simulink model "untitled1"  (R2024b)
settings: Solver=VariableStepAuto  StartTime=0.0  StopTime=0.005  RelTol=1e-3
libraries: simulink x1
settings Model: Creator=valun  LastModifiedBy=valun

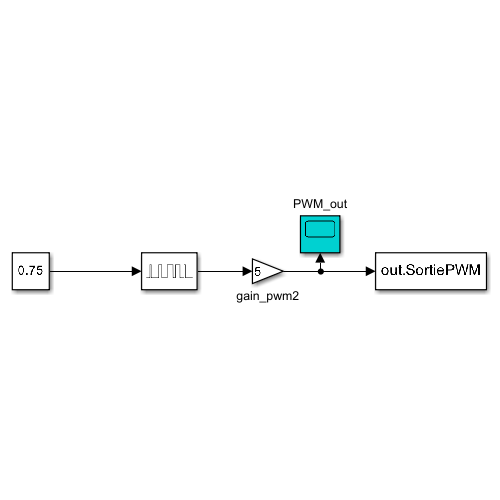
[thumbnail: Simulink's stored preview of the top-level diagram]
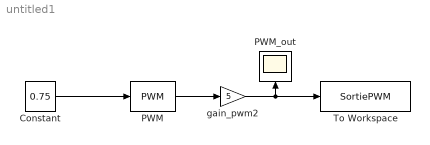
== system untitled1 ==
  Constant : Constant  Value=0.75
  PWM : simulink/Discontinuities/PWM  DisableCoverage=on  Period=0.001  InitialDelay=0  DisallowZeroDutyCycle=off  RunAtFixedTimeIntervals=off  SampleTime=0.1
  PWM_out : Scope
  To Workspace : ToWorkspace  VariableName=SortiePWM  SampleTime=-1
  gain_pwm2 : Gain  Gain=5
  wires:
  gain_pwm2/1 -> PWM_out/1, To Workspace/1
  PWM/1 -> gain_pwm2/1
  Constant/1 -> PWM/1
